simulink model "railway01"  (Simulink 6.5)
settings: Solver=FixedStepDiscrete  StartTime=0.0  StopTime=inf  FixedStep=0.01  RelTol=1e-3
undefined symbols (not defined in the file or in its folder): blocklength
libraries: simulink x10
settings Model: Creator=sja  LastModifiedBy=haf  ExtModeAutoUpdateStatusClock=off
settings DebuggingCC: MultiTaskDSMMsg=warning  MultiTaskCondExecSysMsg=none  StrictBusMsg=None
settings RTWCC: IncludeERTFirstTime=on

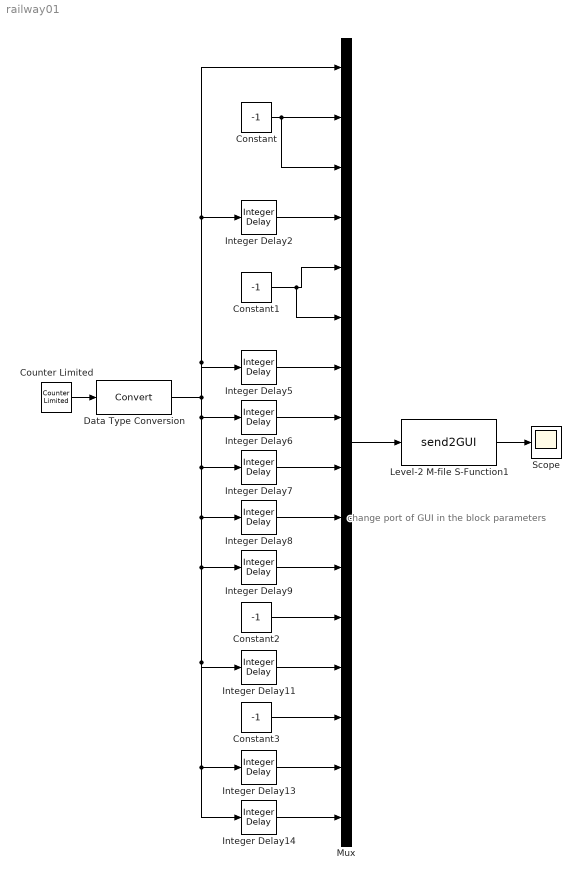
== system railway01 ==
  note: change port of
      | GUI in the block
      | parameters
  Constant{,1..3} (4 alike) : Constant  Value=-1  OutDataType=sfix(16)  ConRadixGroup=Use specified scaling  OutScaling=2^0  SampleTime=inf  FramePeriod=inf
  Counter Limited : simulink/Sources/Counter Limited  SystemSampleTime=-1  uplimit=201  tsamp=-1
  Data Type Conversion : DataTypeConversion
  Integer Delay11 : simulink/Discrete/Integer Delay  vinit=-1  samptime=-1  NumDelays=7*blocklength
  Integer Delay13 : simulink/Discrete/Integer Delay  vinit=-1  samptime=-1  NumDelays=8*blocklength
  Integer Delay14 : simulink/Discrete/Integer Delay  vinit=-1  samptime=-1  NumDelays=9*blocklength
  Integer Delay2 : simulink/Discrete/Integer Delay  vinit=-1  samptime=-1  NumDelays=1*blocklength
  Integer Delay5 : simulink/Discrete/Integer Delay  vinit=-1  samptime=-1  NumDelays=2*blocklength
  Integer Delay6 : simulink/Discrete/Integer Delay  vinit=-1  samptime=-1  NumDelays=3*blocklength
  Integer Delay7 : simulink/Discrete/Integer Delay  vinit=-1  samptime=-1  NumDelays=4*blocklength
  Integer Delay8 : simulink/Discrete/Integer Delay  vinit=-1  samptime=-1  NumDelays=5*blocklength
  Integer Delay9 : simulink/Discrete/Integer Delay  vinit=-1  samptime=-1  NumDelays=6*blocklength
  Level-2 M-file S-Function1 : M-S-Function  FunctionName=send2GUI  Parameters=port,dimensions,sampletime  mask{port=1234, dimensions=0, sampletime=-1}
      mask prompts: port "TCP Port for GUI server"; dimensions "Output Port Dimensions"
      mask help: Interface Block to pass data between the model and a graphical user interface accessed via TCP/IP.
      mask Display:
      | fprintf('GUI INTERFACE\n\n')
      | fprintf(['Port: ' num2str(port)])
  Mux : Mux  Inputs=16
  Scope : Scope
      settings: YMin=0.95  YMax=1.05
  wires:
  Level-2 M-file S-Function1/1 -> Scope/1
  Mux/1 -> Level-2 M-file S-Function1/1
  Counter Limited/1 -> Data Type Conversion/1
  Integer Delay2/1 -> Mux/4
  Integer Delay5/1 -> Mux/7
  Integer Delay6/1 -> Mux/8
  Integer Delay7/1 -> Mux/9
  Integer Delay8/1 -> Mux/10
  Integer Delay9/1 -> Mux/11
  Integer Delay11/1 -> Mux/13
  Integer Delay13/1 -> Mux/15
  Integer Delay14/1 -> Mux/16
  Constant/1 -> Mux/2, Mux/3
  Constant1/1 -> Mux/5, Mux/6
  Constant2/1 -> Mux/12
  Constant3/1 -> Mux/14
  Data Type Conversion/1 -> Integer Delay5/1, Integer Delay2/1, Mux/1, Integer Delay6/1, Integer Delay7/1, Integer Delay8/1, Integer Delay9/1, Integer Delay11/1, Integer Delay13/1, Integer Delay14/1
